simulink model "sgp4test"  (R2023a)
settings: Solver=ode45  StartTime=0.0  StopTime=604800  FixedStep=0.1  MaxStep=1  RelTol=1e-3  EnableMultiTasking=on
libraries: aausat3_lib x2
settings Model: Creator=KFJensen  LastModifiedBy=jacobel-omar
settings SolverCC: AlgebraicLoopSolver=TrustRegion
settings DataIOCC: SaveFormat=Array  SignalLoggingSaveFormat=ModelDataLogs  ReturnWorkspaceOutputs=off
settings OptimizationCC: ExpressionDepthLimit=2147483647  LifeSpan=inf
settings DebuggingCC: UnderspecifiedInitializationDetection=Classic  MergeDetectMultiDrivingBlocksExec=none  SolverPrmCheckMsg=warning  FcnCallInpInsideContextMsg=warning  UnconnectedInputMsg=warning  UnconnectedOutputMsg=warning  UnconnectedLineMsg=warning  StateNameClashWarn=warning  SFUnexpectedBacktrackingDiag=warning  SFNoUnconditionalDefaultTransitionDiag=warning  SFExecutionAtInitializationDiag=none  ArithmeticOperatorsInVariantConditions=warning
settings HardwareCC: ProdBitPerPointer=32  ProdBitPerSizeT=32  ProdBitPerPtrDiffT=32  ProdLargestAtomicFloat=None  ProdIntDivRoundTo=Undefined  ProdEndianess=Unspecified  ProdWordSize=32  ProdHWDeviceType=Generic->Unspecified (assume 32-bit Generic)
settings ModelReferenceCC: PropagateSignalLabelsOutOfModel=off
settings SFSimCC: SimUseLocalCustomCode=off  CustomCodeUndefinedFunction=UseInterfaceOnly
settings RTWCC: RTWUseLocalCustomCode=off
settings CodeAppCC: StateflowObjectComments=on
settings GRTTargetCC: TargetLangStandard=C89/C90 (ANSI)  CombineOutputUpdateFcns=off  GRTInterface=on
settings ConfigComp: CovMetricSettings=dw  CovSaveCumulativeToWorkspaceVar=on  CovSaveSingleToWorkspaceVar=on  CovExternalEMLEnable=off

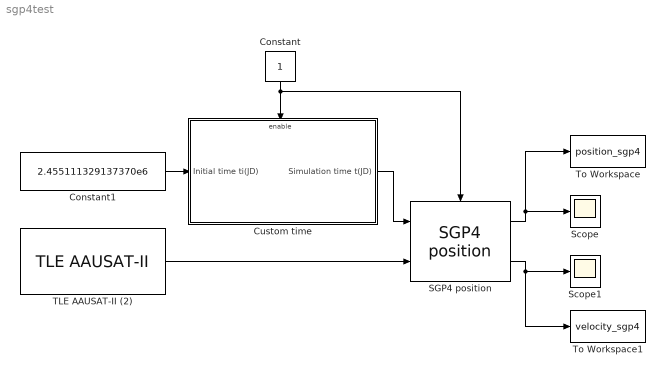
== system sgp4test ==
  Constant : Constant
  Constant1 : Constant  Value=2.455111329137370e6
  Custom time : Subsystem  AncestorBlock=aausat3_lib/Orbit and Ephemeris/Custom time  TreatAsAtomicUnit=on
  SGP4 position : aausat3_lib/Orbit and Ephemeris/SGP4 position  SystemSampleTime=-1  VariantActivationTime=update diagram  Latency=0  AutoFrameSizeCalculation=off
      settings: SourceProductName=AAUSAT3
  Scope : Scope
  Scope1 : Scope
  TLE AAUSAT-II (2) : aausat3_lib/Orbit and Ephemeris/TLE AAUSAT-II  satname='AAUSAT-II'  JulianDay=09321.69542252  xndt2o=0.00000555  xndd6o=0.0  bstar=.76898e-4  xincl=97.9251  xnodeo=24.1597  eo=0.0014245  omegao=254.1774  xmo=105.7862  xno=14.81823818  ts=1
      settings: SourceProductName=AAUSAT3
  To Workspace : ToWorkspace  VariableName=position_sgp4  SampleTime=-1
  To Workspace1 : ToWorkspace  VariableName=velocity_sgp4  SampleTime=-1
  wires:
  Custom time/1(Simulation time t(JD)) -> SGP4 position/1
  Constant/1 -> Custom time/Enable, SGP4 position/Enable
  SGP4 position/1 -> To Workspace/1, Scope/1
  SGP4 position/2 -> Scope1/1, To Workspace1/1
  Constant1/1 -> Custom time/1(Initial time ti(JD))
  TLE AAUSAT-II (2)/1 -> SGP4 position/2

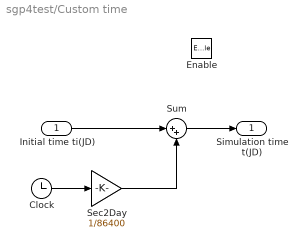
== system sgp4test/Custom time ==
  Initial time ti(JD) : Inport
  Enable : EnablePort
  Clock : Clock
  Sec2Day : Gain  Gain=1/86400  SaturateOnIntegerOverflow=on  OutDataTypeStr=Inherit: Same as input  ParamDataTypeStr=Inherit: Same as input
  Sum : Sum  Inputs=|++
  Simulation time t(JD) : Outport
  wires:
  Initial time ti(JD)/1 -> Sum/1
  Sec2Day/1 -> Sum/2
  Clock/1 -> Sec2Day/1
  Sum/1 -> Simulation time t(JD)/1
